simulink subsystem "GenericAddModulation"  (R2024a)
settings: Solver=VariableStepAuto  StartTime=0.0  StopTime=10.0  RelTol=1e-3
model mask{mod_min=0, mod_max=max_lfo_freq, out_min=0, out_max=max_lfo_freq}
libraries: simulink x1
settings Model: Creator=david  LastModifiedBy=david

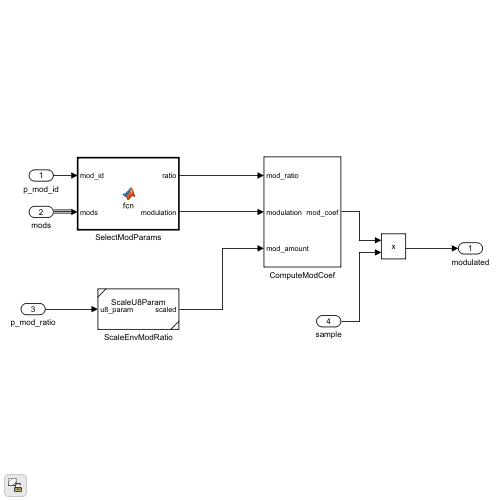
[thumbnail: Simulink's stored preview of the top-level diagram]
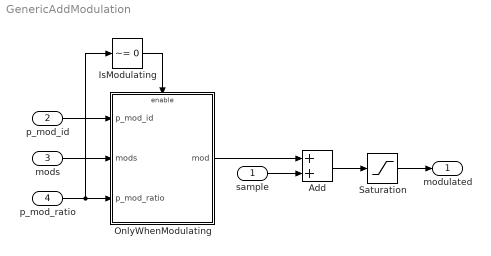
== system GenericAddModulation ==
  sample : Inport
  p_mod_id : Inport  Port=2  OutDataTypeStr=uint8
  mods : Inport  Port=3
  p_mod_ratio : Inport  Port=4
  Add : Sum
  IsModulating : simulink/Logic and Bit Operations/Compare To Zero  relop=~=  OutDataTypeStr=boolean
  OnlyWhenModulating : Subsystem  TreatAsAtomicUnit=on
  Saturation : Saturate  UpperLimit=out_max  LowerLimit=out_min
  modulated : Outport
  wires:
  sample/1 -> Add/2
  Add/1 -> Saturation/1
  Saturation/1 -> modulated/1
  OnlyWhenModulating/1(mod) -> Add/1
  p_mod_id/1 -> OnlyWhenModulating/1(p_mod_id)
  mods/1 -> OnlyWhenModulating/2(mods)
  p_mod_ratio/1 -> OnlyWhenModulating/3(p_mod_ratio), IsModulating/1
  IsModulating/1 -> OnlyWhenModulating/Enable

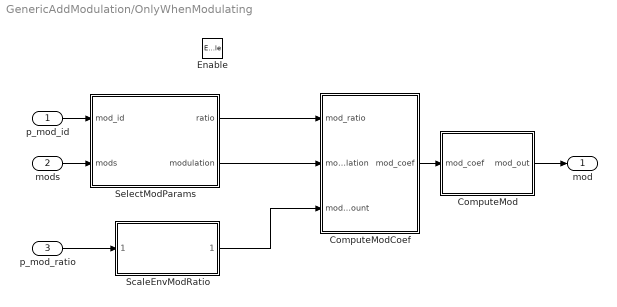
== system GenericAddModulation/OnlyWhenModulating ==
  p_mod_id : Inport  OutDataTypeStr=uint8
  mods : Inport  Port=2
  p_mod_ratio : Inport  Port=3
  Enable : EnablePort
  ComputeMod : Subsystem
  ComputeModCoef : Subsystem
  ScaleEnvModRatio : Subsystem  ReferencedSubsystem=ScaleU8Param
  SelectModParams : MATLAB Function  TreatAsAtomicUnit=on
  mod : Outport  OutputWhenDisabled=reset  InitialOutput=0
  wires:
  p_mod_ratio/1 -> ScaleEnvModRatio/1
  mods/1 -> SelectModParams/2(mods)
  SelectModParams/2(modulation) -> ComputeModCoef/2(modulation)
  ScaleEnvModRatio/1 -> ComputeModCoef/3(mod_amount)
  ComputeModCoef/1(mod_coef) -> ComputeMod/1(mod_coef)
  SelectModParams/1(ratio) -> ComputeModCoef/1(mod_ratio)
  p_mod_id/1 -> SelectModParams/1(mod_id)
  ComputeMod/1(mod_out) -> mod/1

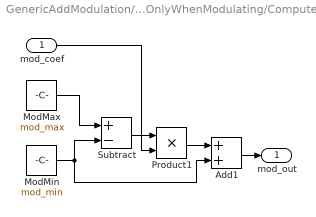
== system GenericAddModulation/OnlyWhenModulating/ComputeMod ==
  mod_coef : Inport
  Add1 : Sum
  ModMax : Constant  Value=mod_max  OutDataTypeStr=single
  ModMin : Constant  Value=mod_min  OutDataTypeStr=single
  Product1 : Product
  Subtract : Sum  Inputs=+-
  mod_out : Outport
  wires:
  ModMin/1 -> Subtract/2, Add1/2
  ModMax/1 -> Subtract/1
  mod_coef/1 -> Product1/2
  Add1/1 -> mod_out/1
  Product1/1 -> Add1/1
  Subtract/1 -> Product1/1

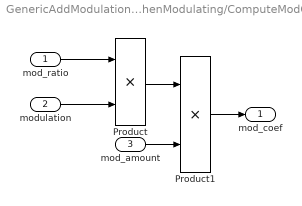
== system GenericAddModulation/OnlyWhenModulating/ComputeModCoef ==
  mod_ratio : Inport
  modulation : Inport  Port=2
  mod_amount : Inport  Port=3
  Product : Product
  Product1 : Product
  mod_coef : Outport
  wires:
  mod_ratio/1 -> Product/1
  Product1/1 -> mod_coef/1
  mod_amount/1 -> Product1/2
  Product/1 -> Product1/1
  modulation/1 -> Product/2

== matlab function GenericAddModulation/OnlyWhenModulating/SelectModParams ==
  data: mod_id input; mods input; ratio output; modulation output
function [ratio, modulation] = fcn(mod_id, mods)
ratio = mods(2 * mod_id + 1);
modulation = mods(2 * mod_id + 2);
